simulink model "PID_Controller"  (R2020a)
settings: Solver=VariableStepAuto  StartTime=0.0  StopTime=120  RelTol=1e-3
PostLoadFcn:
  | m = 1000;
  | b = 50;
  | u = 500;
settings Model: DataDictionary=w2prob3vars.sldd  Creator=Anjali123  LastModifiedBy=Anjali123
settings DataIOCC: SaveOutput=off  SaveTime=off

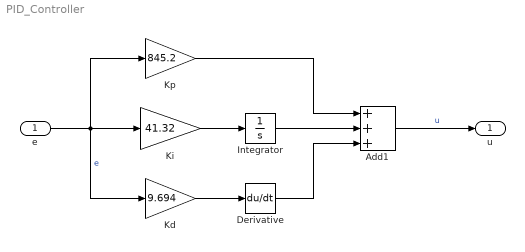
== system PID_Controller ==
  e : Inport  OutDataTypeStr=double  PortDimensions=1  SampleTime=0
  Add1 : Sum  Inputs=+++
  Derivative : Derivative
  Integrator : Integrator
  Kd : Gain  Gain=9.694
  Ki : Gain  Gain=41.32
  Kp : Gain  Gain=845.2
  u : Outport  OutDataTypeStr=double  PortDimensions=1  SampleTime=0
  wires:
  Integrator/1 -> Add1/2
  e/1 -> Kp/1, Ki/1, Kd/1  "e"
  Kd/1 -> Derivative/1
  Add1/1 -> u/1  "u"
  Derivative/1 -> Add1/3
  Kp/1 -> Add1/1
  Ki/1 -> Integrator/1
